simulink model "ControladorDiscreto"  (R2020b)
settings: Solver=FixedStepAuto  StartTime=0.0  StopTime=10.0  FixedStep=0.01  RelTol=1e-3
values from neighbouring files (symbols this model uses):
  k = -2    [Linealizar.m]    (also in routh_hurwitz.m = 2)
  ref = 0.0006    [Linealizar.m]
  u0 = ui(2)    [Linealizar.m]
  x20 = 175    [Curva_linealidad.m]    (also in Linealizar.m = xe(2)+ deltax)
settings Model: Creator=sofia  LastModifiedBy=usuario
settings DataIOCC: SaveOutput=off  SignalLogging=off  DSMLogging=off  SaveTime=off  ReturnWorkspaceOutputs=off

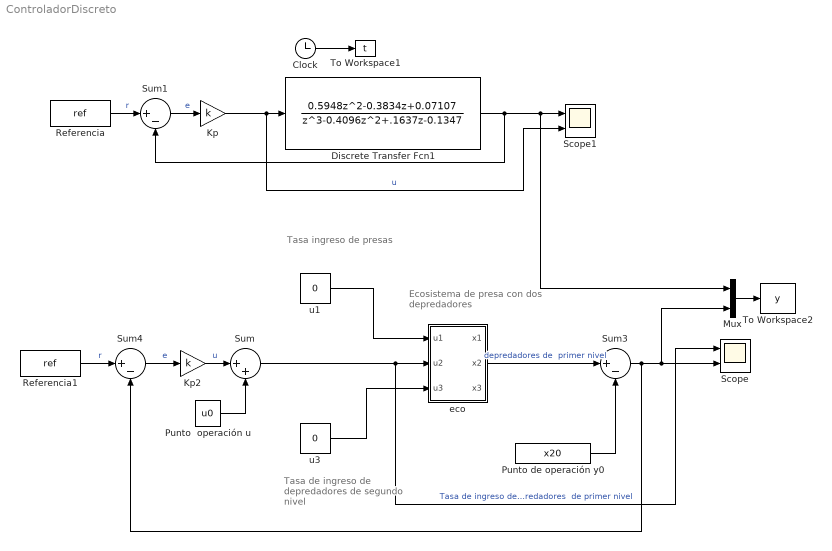
== system ControladorDiscreto ==
  note: Ecosistema de presa
      | con dos depredadores
  note: Tasa ingreso de presas
  note: Tasa de ingreso de depredadores de segundo nivel
  Clock : Clock
  Discrete Transfer Fcn1 : DiscreteTransferFcn  Numerator=[0.5948 -0.3834 0.07107]  Denominator=[1 -0.4096 .1637 -0.1347]
  Kp : Gain  Gain=k
  Kp2 : Gain  Gain=k
  Mux : Mux  Inputs=2
  Punto  operación u : Constant  Value=u0
  Punto de operación y0 : Constant  Value=x20
  Referencia : Constant  Value=ref
  Referencia1 : Constant  Value=ref
  Scope : Scope  NumInputPorts=2
  Scope1 : Scope  NumInputPorts=2
  Sum : Sum  Inputs=|++
  Sum1 : Sum  Inputs=|+-
  Sum3 : Sum  Inputs=|+-
  Sum4 : Sum  Inputs=|+-
  To Workspace1 : ToWorkspace  VariableName=t  SampleTime=-1
  To Workspace2 : ToWorkspace  VariableName=y  SampleTime=-1
  eco : Subsystem  mask(Extensión del modelo Lotka-Volterra para un ecosistema depredador/depredador/presa){ci=[704.569      130.4203      13.04203], ri=[2.84         1.5        0.62], K=8640, ic=[0.02           0        0.03], pc=[0.22           0         0.1]}
      mask prompts: ci "Poblaciones iniciales [x10 x20 x30]"; ri "Tasas de crecimiento intrínseco  [r1 r2 r3]"; K "Capacidad de carga de las presas (K)"; ic "Constantes de interacción [a b c]"; pc "Constantes de proporcionalidad para la capacidad de carga [alpha beta chi]"
      mask help: Sistema de tres ecuaciones diferenciales de primer orden no lineales que describen el comportamiento de un sistema ecológico de tres niveles tróficos: población presa (nivel trófico 1, es depredada por todos), población de depredador de primer nivel (nivel trófico 2, es depredador de la población presa pero también es presa del depredador de segundo nivel) y población de depredador de segundo nivel (nivel trófico 3, es depredador de todos).
      mask init:
      | r1 = ri(1);
      | r2 = ri(2);
      | r3 = ri(3);
      | 
      | 
      | a = ic(1);
      | b = ic(2);
      | c = ic(3);
      | 
      | alpha = pc(1);
      | beta = pc(2);
      | chi = pc(3);
      | 
      | x10 = ci(1);
      | x20 = ci(2);
      | x30 = ci(3);
  u1 : Constant  Value=0
  u3 : Constant  Value=0
  wires:
  Clock/1 -> To Workspace1/1
  u3/1 -> eco/3(u3)
  Kp2/1 -> Sum/1  "u"
  Sum3/1 -> Sum4/2, Mux/2, Scope/2
  Referencia1/1 -> Sum4/1  "r"
  Kp/1 -> Discrete Transfer Fcn1/1, Scope1/2  "u"
  Sum1/1 -> Kp/1  "e"
  Sum4/1 -> Kp2/1  "e"
  Mux/1 -> To Workspace2/1
  Punto de operación y0/1 -> Sum3/2
  eco/2("x2 ") -> Sum3/1  "depredadores de  primer nivel"
  Sum/1 -> Scope/1, eco/2(u2)  "Tasa de ingreso de  depredadores  de primer nivel"
  u1/1 -> eco/1(u1)
  Punto  operación u/1 -> Sum/2
  Discrete Transfer Fcn1/1 -> Sum1/2, Mux/1, Scope1/1
  Referencia/1 -> Sum1/1  "r"

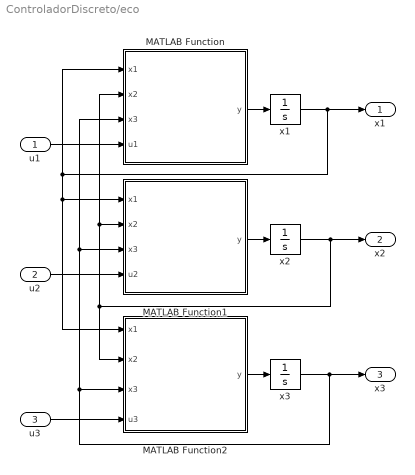
== system ControladorDiscreto/eco ==
  u1 : Inport
  u2 : Inport  Port=2
  u3 : Inport  Port=3
  MATLAB Function : MATLAB Function  TreatAsAtomicUnit=on
  MATLAB Function1 : MATLAB Function  TreatAsAtomicUnit=on
  MATLAB Function2 : MATLAB Function  TreatAsAtomicUnit=on
  x1 : Integrator  InitialCondition=x10  LimitOutput=on  LowerSaturationLimit=0
  x2 : Integrator  InitialCondition=x20  LimitOutput=on  LowerSaturationLimit=0
  x3 : Integrator  InitialCondition=x30  LimitOutput=on  LowerSaturationLimit=0
  "x1 " : Outport
  "x2 " : Outport  Port=2
  "x3 " : Outport  Port=3
  wires:
  x1/1 -> "x1 "/1, MATLAB Function/1(x1), MATLAB Function2/1(x1), MATLAB Function1/1(x1)
  MATLAB Function1/1(y) -> x2/1
  u1/1 -> MATLAB Function/4(u1)
  x3/1 -> "x3 "/1, MATLAB Function1/3(x3), MATLAB Function/3(x3), MATLAB Function2/3(x3)
  MATLAB Function2/1(y) -> x3/1
  x2/1 -> "x2 "/1, MATLAB Function/2(x2), MATLAB Function1/2(x2), MATLAB Function2/2(x2)
  MATLAB Function/1(y) -> x1/1
  u2/1 -> MATLAB Function1/4(u2)
  u3/1 -> MATLAB Function2/4(u3)

== matlab function ControladorDiscreto/eco/MATLAB Function ==
  data: r1 parameter; a parameter; b parameter; K parameter; y output; x1 input; x2 input; x3 input; u1 input
function y = fcn(r1,a,b,K,x1,x2,x3,u1)
y = r1*x1*(1-(x1/K))-a*x1*x2-b*x1*x3 + u1;

== matlab function ControladorDiscreto/eco/MATLAB Function1 ==
  data: r2 parameter; alpha parameter; c parameter; y output; x1 input; x2 input; x3 input; u2 input
function y = fcn(r2,alpha,c,x1,x2,x3,u2)
    term=0;
    if alpha ~=0
        term = (x2/(alpha*x1));
        y = r2*x2*(1-term)-c*x2*x3+u2;
    else
        y = 0;
    end
end

== matlab function ControladorDiscreto/eco/MATLAB Function2 ==
  data: r3 parameter; beta parameter; chi parameter; x1 input; x2 input; x3 input; y output; u3 input
function y = fcn(r3,beta,chi,x1,x2,x3,u3)
    term = 0;
    if not(beta == 0 && chi == 0)
        term = (x3/(beta*x1+chi*x2));
        y = r3*x3*(1-term)+u3;
    else
        y = 0;
    end
end
